simulink subsystem "PowerSystemRef"  (R2022b)
settings: Solver=VariableStepAuto  StartTime=0.0  StopTime=10.0  RelTol=1e-3
settings Model: Creator=drhill  LastModifiedBy=macheson
settings SolverCC: AlgebraicLoopSolver=TrustRegion
settings DebuggingCC: UnconnectedInputMsg=warning  UnconnectedOutputMsg=warning  UnconnectedLineMsg=warning  SFMachineParentedDataDiag=warning
settings ModelReferenceCC: EnableRefExpFcnMdlSchedulingChecks=on
settings RTWCC: DLArmComputeVersion=19.05

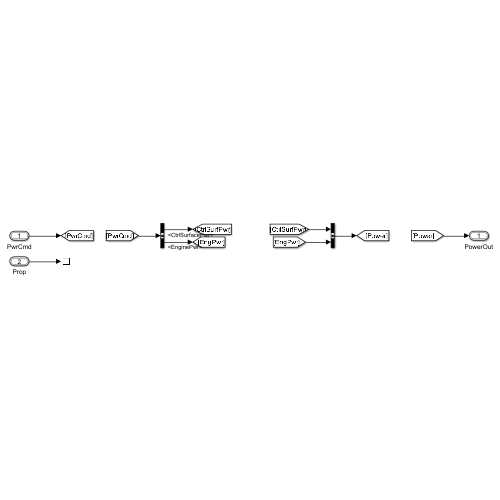
[thumbnail: Simulink's stored preview of the top-level diagram]
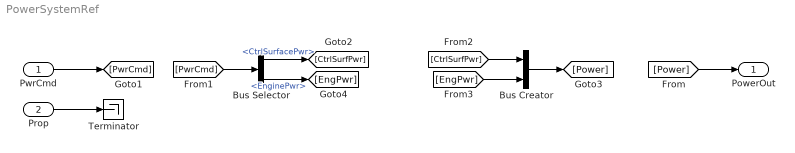
== system PowerSystemRef ==
  PwrCmd : Inport  OutDataTypeStr=Bus: BUS_POWER_SYSTEM_IN
  Prop : Inport  Port=2  OutDataTypeStr=Bus: BUS_PROP_ACTUATOR
  Bus Creator : BusCreator  Inputs=2  OutDataTypeStr=Bus: BUS_POWER_SYSTEM_OUT
  Bus Selector : BusSelector  OutputSignals=CtrlSurfacePwr,EnginePwr
  Terminator : Terminator
  PowerOut : Outport  OutDataTypeStr=Bus: BUS_POWER_SYSTEM_OUT  VectorParamsAs1DForOutWhenUnconnected=off
  wires:
  Prop/1 -> Terminator/1
  Bus Creator/1 -> [Power]
  [Power] -> PowerOut/1
  PwrCmd/1 -> [PwrCmd]
  [PwrCmd] -> Bus Selector/1
  Bus Selector/1 -> [CtrlSurfPwr]  "<CtrlSurfacePwr>"
  Bus Selector/2 -> [EngPwr]  "<EnginePwr>"
  [CtrlSurfPwr] -> Bus Creator/1
  [EngPwr] -> Bus Creator/2
